simulink model "nextpilot_mc_simulation"  (R2024b)
settings: Solver=VariableStepAuto  StartTime=0.0  StopTime=10.0  RelTol=1e-3
settings Model: DataDictionary=nextpilot_datadict.sldd  Creator=CETCA  LastModifiedBy=CETCA

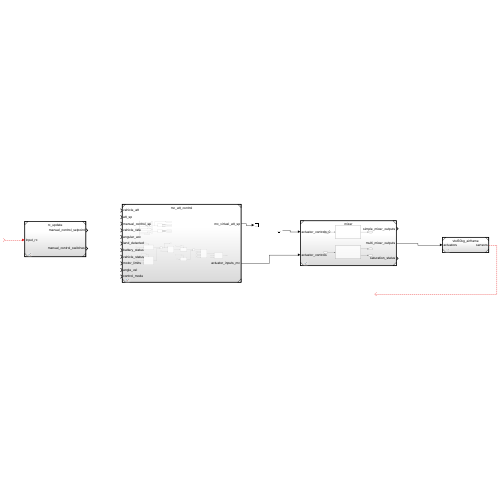
[thumbnail: Simulink's stored preview of the top-level diagram]
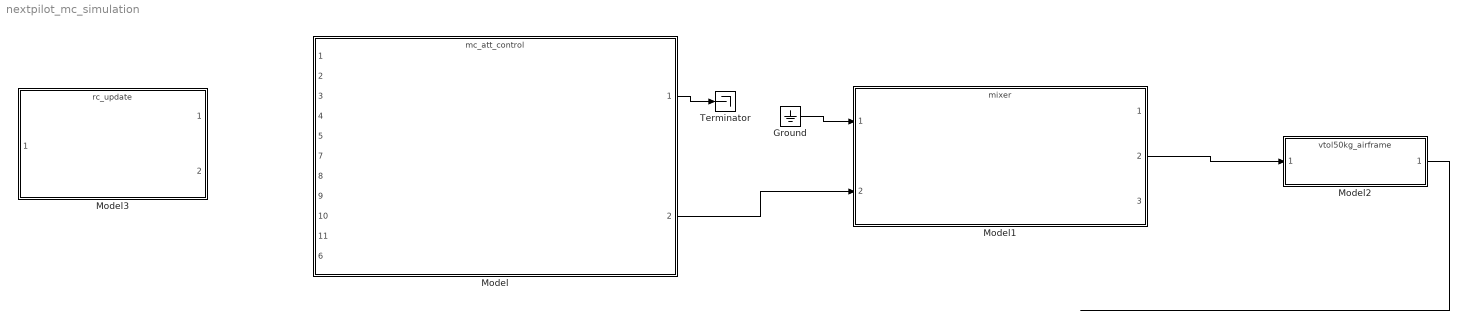
== system nextpilot_mc_simulation ==
  Ground : Ground
  Model : ModelReference  ModelNameDialog=mc_att_control.slx  SimulationMode=Normal  ModelReferenceVersion=1.1321
      settings: PortSchema="{\"entries\":[{\"content\":{\"sides\":[{\"content\":{\"connectorIds\":[\"In1\",\"In2\",\"In3\",\"In4\",\"In5\",\"In7\",\"In8\",\"In9\",\"In10\",\"In11\",\"In6\"]},\"type\":\"ConnectorPlacement.EquallySpacedRectSide\",\"uuid\":\"8fc460c4-4bb1-4c4a-bfc6-ff4de11260b5\"},{\"content\":{\"connectorIds\":[\"Out1\",\"Out2\"],\"side\":\"RIGHT\"},\"type\":\"ConnectorPlacement.EquallySpacedRectSide\",\"uuid\":\"a02b17a1-94e6-4f9f-8165-de6905fde42d\"},{\"content\":{\"side\":\"TOP\"},\"type\":\"ConnectorPlacement.EquallySpacedRectSide\",\"uuid\":\"b1023124-14fc-410d-b667-33d4ec6bc303\"}]},\"type\":\"ConnectorPlacement.EquallySpacedConnector\",\"uuid\":\"199f1363-2c7e-4a0b-982e-23295f2bc331\"}],\"packageUris\":[\"http://schema.mathworks.com/mf0/Connector/R2020b\"],\"version\":\"1.0\"}"
  Model1 : ModelReference  ModelNameDialog=mixer.slx  SimulationMode=Normal  ModelReferenceVersion=8.0
  Model2 : ModelReference  ModelNameDialog=vtol50kg_airframe.slx  SimulationMode=Normal  ModelReferenceVersion=5.276
  Model3 : ModelReference  ModelNameDialog=rc_update.slx  SimulationMode=Normal  ModelReferenceVersion=8.36
  Terminator : Terminator
  wires:
  Ground/1 -> Model1/1
  Model/1 -> Terminator/1
  Model/2 -> Model1/2
  Model1/2 -> Model2/1
  Model2/1 -> ?
  ? -> Model3/1
